simulink model "RLC_policy"  (R2019b)
settings: Solver=VariableStepAuto  StartTime=0.0  StopTime=10  FixedStep=0.1  RelTol=1e-3
libraries: ctrlSharedLib x1
settings Model: Creator=PC2018  LastModifiedBy=PC2018

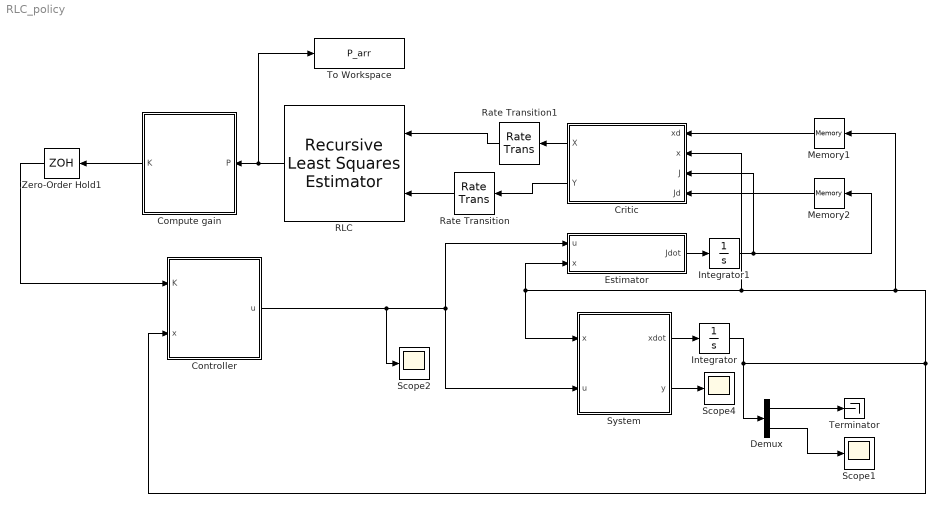
== system RLC_policy ==
  Compute gain : MATLAB Function  TreatAsAtomicUnit=on
  "Controller " : MATLAB Function  TreatAsAtomicUnit=on
  "Critic " : MATLAB Function  TreatAsAtomicUnit=on
  Demux : Demux  Outputs=2
  "Estimator " : MATLAB Function  TreatAsAtomicUnit=on
  Integrator : Integrator  InitialCondition=[5;0]
  Integrator1 : Integrator  InitialCondition=1
  Memory1 : Memory  InitialCondition=[3;0]
  Memory2 : Memory  InitialCondition=20
  RLC : ctrlSharedLib/Recursive Least Squares Estimator  InitialEstimateSource=Internal  InitialParameterData=[0 0 0 0]  P0=1e4  InitialRegressors=0  InitialOutputs=0  History=Infinite  WindowLength=200  EstimationMethod=Forgetting Factor  AdaptationParameter=1  HasTimeVaryingAdaptationParameter=off  NormalizationBias=eps  OutputError=off  OutputP=off  AddEnablePort=off  InputProcessing=Sample-based  Ts=0.01
      settings: SourceProductName=Control System Toolbox  SourceProductBaseCode=CT
  Rate Transition : RateTransition  OutPortSampleTime=0.01
  Rate Transition1 : RateTransition  OutPortSampleTime=0.01
  Scope1 : Scope
  Scope2 : Scope
  Scope4 : Scope
  System : MATLAB Function  TreatAsAtomicUnit=on
  Terminator : Terminator
  To Workspace : ToWorkspace  VariableName=P_arr  SampleTime=-1
  Zero-Order Hold1 : ZeroOrderHold  SampleTime=-1
  wires:
  Integrator1/1 -> Memory2/1, "Critic "/3(J)
  System/1(xdot) -> Integrator/1
  "Controller "/1(u) -> Scope2/1, System/2(u), "Estimator "/1(u)
  Demux/2 -> Scope1/1
  Integrator/1 -> Demux/1, "Critic "/2(x), System/1(x), "Estimator "/2(x), Memory1/1, "Controller "/2(x)
  Memory1/1 -> "Critic "/1(xd)
  "Estimator "/1(Jdot) -> Integrator1/1
  Demux/1 -> Terminator/1
  Memory2/1 -> "Critic "/4(Jd)
  System/2(y) -> Scope4/1
  "Critic "/2(Y) -> Rate Transition/1
  "Critic "/1(X) -> Rate Transition1/1
  RLC/1 -> To Workspace/1, Compute gain/1(P)
  Compute gain/1(K) -> Zero-Order Hold1/1
  Zero-Order Hold1/1 -> "Controller "/1(K)
  Rate Transition1/1 -> RLC/1
  Rate Transition/1 -> RLC/2

== matlab function RLC_policy/Estimator  ==
  data: u input; x input; Jdot output
function Jdot = fcn(u,x)
%Cost function evaluation


Q = [1 0;0 1];
R = 1;
alp = 0.1;



Jdot = x'*Q*x + u'*R*u;

== matlab function RLC_policy/System ==
  data: x input; u input; xdot output; y output
function [xdot,y] = fcn(x,u)

B = [0;1];
A = [0 1;-3 -2];
C = [1 0];


xdot = A*x + B*u;
y = C*x;

== matlab function RLC_policy/Critic  ==
  data: X output; xd input; x input; J input; Y output; Jd input
function [X,Y] = fcn(xd,x,J,Jd)

xd1 = x(1)^2;
xd2 = x(1)*x(2);
xd3 = x(2)*x(1);
xd4 = x(2)^2;

xn1 = xd(1)^2;
xn2 = xd(1)*xd(2);
xn3 = xd(2)*xd(1);
xn4 = xd(2)^2;

x1 = [xd1;xd2;xd3;xd4];
x2 = [xn1;xn2;xn3;xn4];

X = (x2 - x1);
Y = (J-Jd);

== matlab function RLC_policy/Controller  ==
  data: K input; x input; u output
function u = fcn(K, x)
u = 0;

%ddot =
alp = 0.1;
e = [alp^2 alp^2];

u = -K*x;

== matlab function RLC_policy/Compute gain ==
  data: P input; K output
function K = fcn(P)
K = [0 0];
Pi = [0 0;0 0];

B = [0;1];

p1 = P(1);
p12 = P(2)/2;
p21 = P(3)/2;
p2 = P(4);


Pi = [p1, p12;p21, p2];

K = B'*Pi;
